simulink model "rolingroad"  (R2015a)
settings: Solver=ode45  SolverMode=SingleTasking  StartTime=0.0  StopTime=10.0  FixedStep=0.0000001  RelTol=1e-1
libraries: simulink x1
settings Model: Creator=jonathan  LastModifiedBy=jonathan
settings SolverCC: ConsecutiveZCsStepRelTol=100*128*eps  MaxConsecutiveMinStep=100  AutoInsertRateTranBlk=on
settings DataIOCC: ReturnWorkspaceOutputs=on
settings DebuggingCC: ReadBeforeWriteMsg=DisableAll  WriteAfterWriteMsg=DisableAll  WriteAfterReadMsg=DisableAll  MultiTaskDSMMsg=none  ParameterDowncastMsg=warning  ParameterOverflowMsg=warning
settings ModelReferenceCC: UpdateModelReferenceTargets=IfOutOfDate
settings SFSimCC: SFSimEcho=off

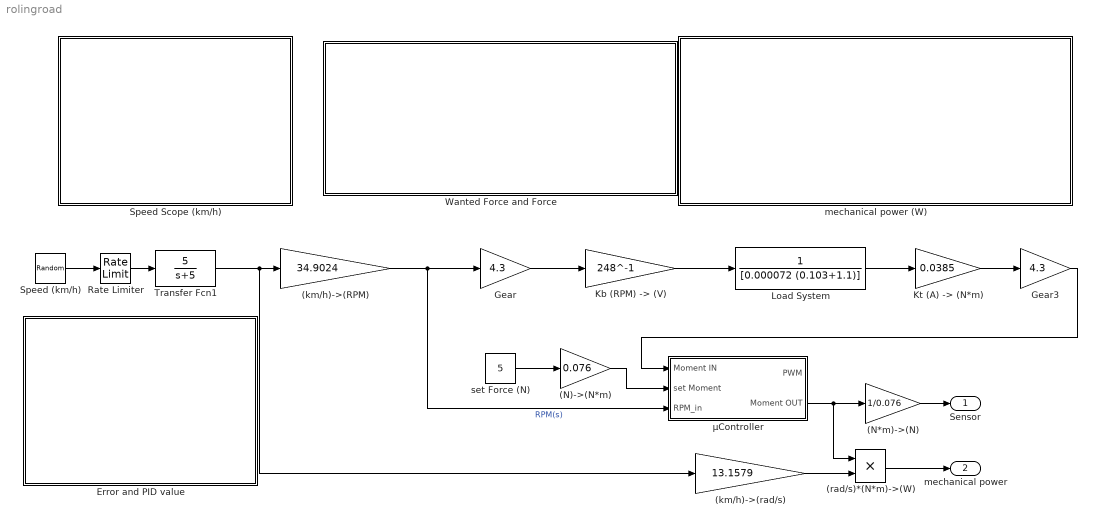
== system rolingroad ==
  (N)->(N*m) : Gain  Gain=0.076
  (N*m)->(N) : Gain  Gain=1/0.076
  (km/h)->(RPM) : Gain  Gain=34.9024
  (km/h)->(rad/s) : Gain  Gain=13.1579
  (rad/s)*(N*m)->(W) : Product
  Error and PID value : Subsystem  DialogController=hmiCreateDDGDialog  IsWebBlock=on  mask(MathWorksWebBlock){webBlockId=e8d74390-8b58-4fce-8b2e-89b837e7f5d5, webBlockType=sdiscope, ShowInitialText=on, HMISrcModelName=rolingroad}
      mask prompts: webBlockId "WebBlock Id"; webBlockType "WebBlock Type"; HMISrcModelName "Source Model"
      mask Help: helpview([docroot '/mapfiles/simulink.map'], 'hmi_scope')
      mask Display:
      | if strcmp(get_param(bdroot(gcb),'BlockDiagramType'), 'library')
      |     image([(matlabroot) '/toolbox/simulink/hmi/icons/DashboardScope.png']);
      | end
  Gear : Gain  Gain=4.3
  Gear3 : Gain  Gain=4.3
  "Kb (RPM) -> (V)" : Gain  Gain=248^-1
  "Kt (A) -> (N*m)" : Gain  Gain=0.0385
  Load System : TransferFcn  Denominator=[0.000072 (0.103+1.1)]
  Rate Limiter : RateLimiter  RisingSlewLimit=10  FallingSlewLimit=-10
  Speed (km/h) : RandomNumber  Mean=24.8  Variance=4  SampleTime=1
  Speed Scope (km/h) : Subsystem  DialogController=hmiCreateDDGDialog  IsWebBlock=on  mask(MathWorksWebBlock){webBlockId=bf6427f6-4289-4f73-813a-1227a3c476fa, webBlockType=sdiscope, ShowInitialText=on, HMISrcModelName=rolingroad}
      mask prompts: webBlockId "WebBlock Id"; webBlockType "WebBlock Type"; HMISrcModelName "Source Model"
      mask Help: helpview([docroot '/mapfiles/simulink.map'], 'hmi_scope')
      mask Display:
      | if strcmp(get_param(bdroot(gcb),'BlockDiagramType'), 'library')
      |     image([(matlabroot) '/toolbox/simulink/hmi/icons/DashboardScope.png']);
      | end
  Transfer Fcn1 : TransferFcn  Numerator=[5]  Denominator=[1 5]
  Wanted Force and Force : Subsystem  DialogController=hmiCreateDDGDialog  IsWebBlock=on  mask(MathWorksWebBlock){webBlockId=7bd36063-daa1-4e14-a4f8-08fe91d46a67, webBlockType=sdiscope, ShowInitialText=on, HMISrcModelName=rolingroad}
      mask prompts: webBlockId "WebBlock Id"; webBlockType "WebBlock Type"; HMISrcModelName "Source Model"
      mask Help: helpview([docroot '/mapfiles/simulink.map'], 'hmi_scope')
      mask Display:
      | if strcmp(get_param(bdroot(gcb),'BlockDiagramType'), 'library')
      |     image([(matlabroot) '/toolbox/simulink/hmi/icons/DashboardScope.png']);
      | end
  mechanical power (W) : Subsystem  DialogController=hmiCreateDDGDialog  IsWebBlock=on  mask(MathWorksWebBlock){webBlockId=78a41241-16df-4e3b-8e87-14d564f6b89d, webBlockType=sdiscope, ShowInitialText=on, HMISrcModelName=rolingroad}
      mask prompts: webBlockId "WebBlock Id"; webBlockType "WebBlock Type"; HMISrcModelName "Source Model"
      mask Help: helpview([docroot '/mapfiles/simulink.map'], 'hmi_scope')
      mask Display:
      | if strcmp(get_param(bdroot(gcb),'BlockDiagramType'), 'library')
      |     image([(matlabroot) '/toolbox/simulink/hmi/icons/DashboardScope.png']);
      | end
  set Force (N) : Constant  Value=5
  µController : Subsystem
  Sensor : Outport
  mechanical power : Outport  Port=2
  wires:
  set Force (N)/1 -> (N)->(N*m)/1
  (km/h)->(RPM)/1 -> µController/3(RPM_in), Gear/1  "RPM(s)"
  µController/2(Moment OUT) -> (N*m)->(N)/1, (rad/s)*(N*m)->(W)/1
  Speed (km/h)/1 -> Rate Limiter/1
  Rate Limiter/1 -> Transfer Fcn1/1
  Transfer Fcn1/1 -> (km/h)->(RPM)/1, (km/h)->(rad/s)/1
  Gear/1 -> "Kb (RPM) -> (V)"/1
  (N*m)->(N)/1 -> Sensor/1
  "Kt (A) -> (N*m)"/1 -> Gear3/1
  Load System/1 -> "Kt (A) -> (N*m)"/1
  Gear3/1 -> µController/1(Moment IN)
  (N)->(N*m)/1 -> µController/2(set Moment)
  "Kb (RPM) -> (V)"/1 -> Load System/1
  (rad/s)*(N*m)->(W)/1 -> mechanical power/1
  (km/h)->(rad/s)/1 -> (rad/s)*(N*m)->(W)/2

== system rolingroad/Error and PID value ==

== system rolingroad/Speed Scope (km//h) ==

== system rolingroad/Wanted Force and Force ==

== system rolingroad/mechanical power (W) ==

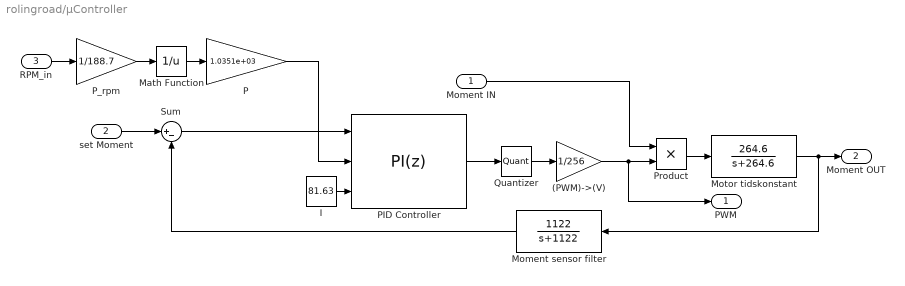
== system rolingroad/µController ==
  Moment IN : Inport
  set Moment : Inport  Port=2
  RPM_in : Inport  Port=3
  (PWM)->(V) : Gain  Gain=1/256
  I : Constant  Value=81.63
  Math Function : Math  Operator=reciprocal  OutputSignalType=real  OutMin=[0]  OutMax=[188.7]  SaturateOnIntegerOverflow=on
  Moment sensor filter : TransferFcn  Numerator=[1122]  Denominator=[1 1122]
  Motor tidskonstant : TransferFcn  Numerator=[264.6]  Denominator=[1 264.6]  AbsoluteTolerance=50
  P : Gain  Gain=1.0351e+03
  PID Controller : simulink/Continuous/PID Controller  Controller=PI  TimeDomain=Discrete-time  SampleTime=1.8382e-04  IntegratorMethod=Forward Euler  FilterMethod=Forward Euler  Form=Ideal  UseFilter=off  ControllerParametersSource=external  P=1000  I=81.6  D=-0.00741521132146646  N=107.889000574029  InitialConditionSource=internal  InitialConditionForIntegrator=0  InitialConditionForFilter=0  ExternalReset=none  LimitOutput=on  UpperSaturationLimit=256  LowerSaturationLimit=0  LinearizeAsGain=off  AntiWindupMode=clamping  Kb=1  TrackingMode=off  Kt=1  PParamMin=[]  PParamMax=[]  IParamMin=[]  IParamMax=[]  DParamMin=[]  DParamMax=[]  NParamMin=[]  NParamMax=[]  KbParamMin=[]  KbParamMax=[]  KtParamMin=[]  KtParamMax=[]  POutMin=[]  POutMax=[]  IOutMin=[]  IOutMax=[]  DOutMin=[]  DOutMax=[]  NOutMin=[]  NOutMax=[]  KbOutMin=[]  KbOutMax=[]  KtOutMin=[]  KtOutMax=[]  IntegratorOutMin=[]  IntegratorOutMax=[]  FilterOutMin=[]  FilterOutMax=[]  SumOutMin=[]  SumOutMax=[]  SumI1OutMin=[]  SumI1OutMax=[]  SumI2OutMin=[]  SumI2OutMax=[]  SumI3OutMin=[]  SumI3OutMax=[]  SumDOutMin=[]  SumDOutMax=[]  SaturationOutMin=[]  SaturationOutMax=[]  IntegratorContinuousStateAttributes=''  IntegratorStateMustResolveToSignalObject=off  IntegratorRTWStateStorageClass=Auto  FilterContinuousStateAttributes=''  FilterStateMustResolveToSignalObject=off  FilterRTWStateStorageClass=Auto  DifferentiatorICPrevScaledInput=0  DifferentiatorOutMin=[]  DifferentiatorOutMax=[]
  P_rpm : Gain  Gain=1/188.7
  Product : Product
  Quantizer : Quantizer  QuantizationInterval=1
  Sum : Sum  Inputs=|+-
  PWM : Outport
  Moment OUT : Outport  Port=2
  wires:
  set Moment/1 -> Sum/1
  Quantizer/1 -> (PWM)->(V)/1
  Product/1 -> Motor tidskonstant/1
  (PWM)->(V)/1 -> Product/2, PWM/1
  Motor tidskonstant/1 -> Moment OUT/1, Moment sensor filter/1
  Moment IN/1 -> Product/1
  RPM_in/1 -> P_rpm/1
  P_rpm/1 -> Math Function/1
  Math Function/1 -> P/1
  Moment sensor filter/1 -> Sum/2
  Sum/1 -> PID Controller/1
  I/1 -> PID Controller/3
  P/1 -> PID Controller/2
  PID Controller/1 -> Quantizer/1
